simulink model "Grua"  (R2024b)
settings: Solver=VariableStepAuto  StartTime=0.0  StopTime=50.0  RelTol=1e-3
values from neighbouring files (symbols this model uses):
  A1 = [0 0 1 0; 0 0 0 1; 0 0 carrito_ss.A(2,2) 0; 0 pendulo_ss.A(2,1) 0 pendulo_ss.A(2,2)]    [Grua_Pendulo_Control.m]    (also in grua.mat = [0 0 0 0 0 0 0 -35.3130710133 1 0 -9.69067245938 0 ... (16 e)
  B1 = [0; pendulo_ss.B(1); carrito_ss.B(2); pendulo_ss.B(2)]    [Grua_Pendulo_Control.m]    (also in grua.mat = [0 -0.296894785399 0.236071876692 -1.46592019656])
  C = [1 0 0 0]    [Grua_Pendulo_Control.m]    (also in grua.mat)
  K = Ks(1:4)    [Grua_Pendulo_Control.m]    (also in grua.mat = [11.2779924086 -1.98610202692 -5.28014178733 -2.15028681626])
  K_q = Kq(1:4)    [Grua_Pendulo_Control.m]    (also in grua.mat = [50.0170795212 -5.53286476625 6.72231103684 -0.384358946683])
  Ki = -Ks(5)    [Grua_Pendulo_Control.m]    (also in grua.mat = 4.13832170273)
  Ki_q = -Kq(5)    [Grua_Pendulo_Control.m]    (also in grua.mat = 20)
libraries: simulink x5, slpidlib x3
settings Model: Creator=nagel  LastModifiedBy=nagel

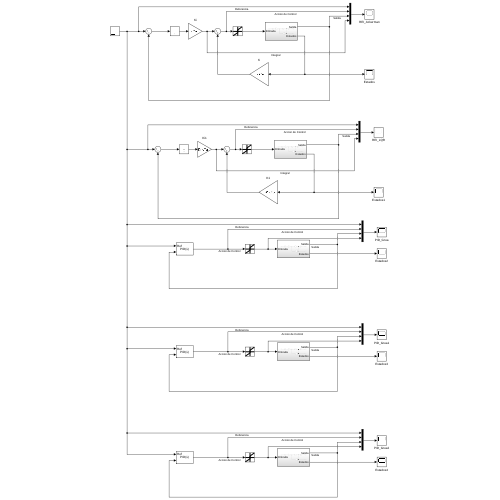
[thumbnail: Simulink's stored preview of the top-level diagram]
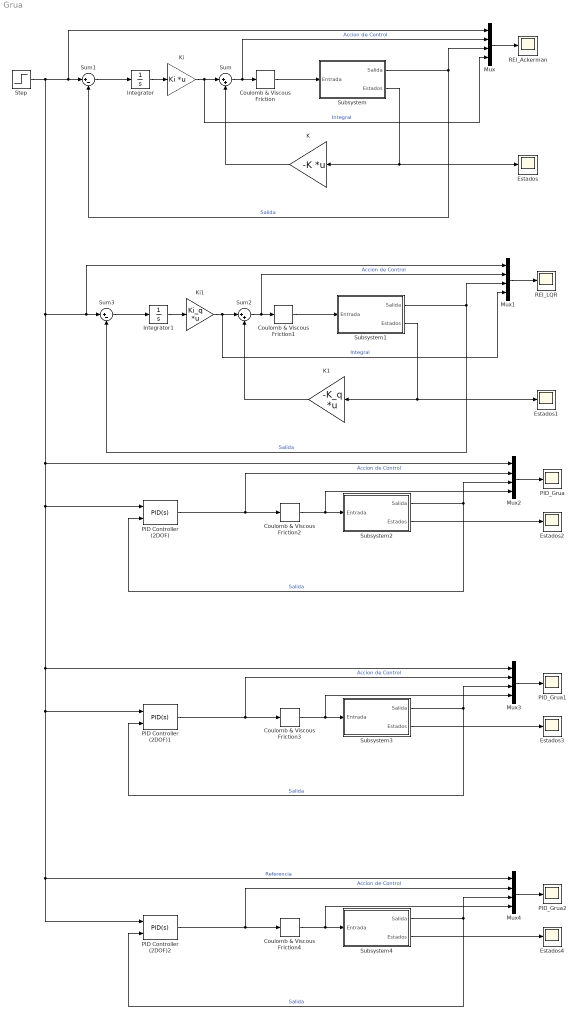
== system Grua ==
  Coulomb & Viscous Friction{,1..4} (5 alike) : simulink/Discontinuities/Coulomb & Viscous Friction  offset=[0.4]  gain=1
  Estados{,1..4} (5 alike) : Scope
  Integrator : Integrator
  Integrator1 : Integrator
  K : Gain  Gain=-K  Multiplication=Matrix(K*u)
  K1 : Gain  Gain=-K_q  Multiplication=Matrix(K*u)
  Ki : Gain  Gain=Ki  Multiplication=Matrix(K*u)
  Ki1 : Gain  Gain=Ki_q  Multiplication=Matrix(K*u)
  Mux{,1..4} (5 alike) : Mux
  PID Controller (2DOF) : slpidlib/PID Controller (2DOF)  Controller=PID  Form=Parallel  TimeDomain=Continuous-time  UseExternalTs=off  SampleTime=-1  IntegratorMethod=Forward Euler  FilterMethod=Forward Euler  ControllerParametersSource=internal  P=30.1626  I=0.3867  UseKiTs=off  D=0  UseExternalDerivativeSource=off  N=0  UseFilter=on  b=1  c=1  TunerSelectOption=Transfer Function Based (PID Tuner App)  InitialConditionSource=internal  InitialConditionForIntegrator=0  InitialConditionForFilter=0  DifferentiatorICPrevScaledInput=0  ExternalReset=none  TrackingMode=off  Kt=1  LimitOutput=off  SatLimitsSource=internal  UpperSaturationLimit=inf  LowerSaturationLimit=-inf  LinearizeAsGain=on  AntiWindupMode=none  Kb=1  LimitIntegrator=off  UpperIntegratorSaturationLimit=inf  LowerIntegratorSaturationLimit=-inf  POutMin=[]  POutMax=[]  IOutMin=[]  IOutMax=[]  DOutMin=[]  DOutMax=[]  NOutMin=[]  NOutMax=[]  bOutMin=[]  bOutMax=[]  cOutMin=[]  cOutMax=[]  SumOutMin=[]  SumOutMax=[]  SaturationOutMin=[]  SaturationOutMax=[]  PParamMin=[]  PParamMax=[]  IParamMin=[]  IParamMax=[]  DParamMin=[]  DParamMax=[]  NParamMin=[]  NParamMax=[]  bParamMin=[]  bParamMax=[]  cParamMin=[]  cParamMax=[]  KbParamMin=[]  KbParamMax=[]  KtParamMin=[]  KtParamMax=[]  KbOutMin=[]  KbOutMax=[]  KtOutMin=[]  KtOutMax=[]  IntegratorOutMin=[]  IntegratorOutMax=[]  FilterOutMin=[]  FilterOutMax=[]  SumI1OutMin=[]  SumI1OutMax=[]  SumI2OutMin=[]  SumI2OutMax=[]  SumI3OutMin=[]  SumI3OutMax=[]  SumI4OutMin=[]  SumI4OutMax=[]  SumDOutMin=[]  SumDOutMax=[]  Sum1OutMin=[]  Sum1OutMax=[]  Sum2OutMin=[]  Sum2OutMax=[]  Sum3OutMin=[]  Sum3OutMax=[]  DifferentiatorOutMin=[]  DifferentiatorOutMax=[]  FilterDiffOutCoefMin=[]  FilterDiffOutCoefMax=[]  ReciprocalOutMin=[]  ReciprocalOutMax=[]  SumDenOutMin=[]  SumDenOutMax=[]  SumNumOutMin=[]  SumNumOutMax=[]  DivideOutMin=[]  DivideOutMax=[]  UdiffTsProdOutMin=[]  UdiffTsProdOutMax=[]  NTsProdOutMin=[]  NTsProdOutMax=[]  UintegralTsProdOutMin=[]  UintegralTsProdOutMax=[]  UngainTsProdOutMin=[]  UngainTsProdOutMax=[]  ClampingZeroOutDataTypeStr=Inherit: Inherit via back propagation  ClampingZeroOutMin=[]  ClampingZeroOutMax=[]  FilterDenConstantOutDataTypeStr=Inherit: Inherit via back propagation  FilterDenConstantOutMin=[]  FilterDenConstantOutMax=[]  PCopyOutDataTypeStr=Inherit: Inherit via back propagation  PCopyOutMin=[]  PCopyOutMax=[]  NCopyOutDataTypeStr=Inherit: Inherit via back propagation  NCopyOutMin=[]  NCopyOutMax=[]  IntegratorContinuousStateAttributes=''  IntegratorStateMustResolveToSignalObject=off  IntegratorRTWStateStorageClass=Auto  FilterContinuousStateAttributes=''  FilterStateMustResolveToSignalObject=off  FilterRTWStateStorageClass=Auto  ParallelPVariant=InternalParameters  IdealPVariant=Disabled  IVariant=InternalParameters  DVariant=InternalParameters  bVariant=InternalParameters  cVariant=InternalParameters  IntegratorVariant=Continuous  SatVariant=Disabled  AWVariant=Passthrough  PCopyVariant=Disabled  TRVariant=Disabled  FdbkBlocksVariant=Forward  IdealPFdbkVariant=Disabled  SatFdbkVariant=Disabled  DerivativeFilterVariant=ContFilter  NVariant=InternalParameters  NCopyVariant=Disabled  FilterICVariant=InternalICsFilter  IntegratorICVariant=InternalICs  ExternalResetVariant=Disabled  TRSumVariant=Passthrough  SumFdbkVariant=Disabled  SumVariant=Sum_PID  TsampFilterVariant=InternalTs  TsampNgainVariant=Passthrough  TsampIntegralVariant=Disabled_SignalSpec  ExternalSaturationOutDataTypeStr=Inherit: Same as second input  DerivativeSourceVariant=ErrorSignal  PreIntVariant=InternalPreInt
  PID Controller (2DOF)1 : slpidlib/PID Controller (2DOF)  Controller=PID  Form=Parallel  TimeDomain=Continuous-time  UseExternalTs=off  SampleTime=-1  IntegratorMethod=Forward Euler  FilterMethod=Forward Euler  ControllerParametersSource=internal  P=16.75  I=95.23  UseKiTs=off  D=38.239  UseExternalDerivativeSource=off  N=270.27  UseFilter=on  b=1  c=1  TunerSelectOption=Transfer Function Based (PID Tuner App)  InitialConditionSource=internal  InitialConditionForIntegrator=0  InitialConditionForFilter=0  DifferentiatorICPrevScaledInput=0  ExternalReset=none  TrackingMode=off  Kt=1  LimitOutput=off  SatLimitsSource=internal  UpperSaturationLimit=inf  LowerSaturationLimit=-inf  LinearizeAsGain=on  AntiWindupMode=none  Kb=1  LimitIntegrator=off  UpperIntegratorSaturationLimit=inf  LowerIntegratorSaturationLimit=-inf  POutMin=[]  POutMax=[]  IOutMin=[]  IOutMax=[]  DOutMin=[]  DOutMax=[]  NOutMin=[]  NOutMax=[]  bOutMin=[]  bOutMax=[]  cOutMin=[]  cOutMax=[]  SumOutMin=[]  SumOutMax=[]  SaturationOutMin=[]  SaturationOutMax=[]  PParamMin=[]  PParamMax=[]  IParamMin=[]  IParamMax=[]  DParamMin=[]  DParamMax=[]  NParamMin=[]  NParamMax=[]  bParamMin=[]  bParamMax=[]  cParamMin=[]  cParamMax=[]  KbParamMin=[]  KbParamMax=[]  KtParamMin=[]  KtParamMax=[]  KbOutMin=[]  KbOutMax=[]  KtOutMin=[]  KtOutMax=[]  IntegratorOutMin=[]  IntegratorOutMax=[]  FilterOutMin=[]  FilterOutMax=[]  SumI1OutMin=[]  SumI1OutMax=[]  SumI2OutMin=[]  SumI2OutMax=[]  SumI3OutMin=[]  SumI3OutMax=[]  SumI4OutMin=[]  SumI4OutMax=[]  SumDOutMin=[]  SumDOutMax=[]  Sum1OutMin=[]  Sum1OutMax=[]  Sum2OutMin=[]  Sum2OutMax=[]  Sum3OutMin=[]  Sum3OutMax=[]  DifferentiatorOutMin=[]  DifferentiatorOutMax=[]  FilterDiffOutCoefMin=[]  FilterDiffOutCoefMax=[]  ReciprocalOutMin=[]  ReciprocalOutMax=[]  SumDenOutMin=[]  SumDenOutMax=[]  SumNumOutMin=[]  SumNumOutMax=[]  DivideOutMin=[]  DivideOutMax=[]  UdiffTsProdOutMin=[]  UdiffTsProdOutMax=[]  NTsProdOutMin=[]  NTsProdOutMax=[]  UintegralTsProdOutMin=[]  UintegralTsProdOutMax=[]  UngainTsProdOutMin=[]  UngainTsProdOutMax=[]  ClampingZeroOutDataTypeStr=Inherit: Inherit via back propagation  ClampingZeroOutMin=[]  ClampingZeroOutMax=[]  FilterDenConstantOutDataTypeStr=Inherit: Inherit via back propagation  FilterDenConstantOutMin=[]  FilterDenConstantOutMax=[]  PCopyOutDataTypeStr=Inherit: Inherit via back propagation  PCopyOutMin=[]  PCopyOutMax=[]  NCopyOutDataTypeStr=Inherit: Inherit via back propagation  NCopyOutMin=[]  NCopyOutMax=[]  IntegratorContinuousStateAttributes=''  IntegratorStateMustResolveToSignalObject=off  IntegratorRTWStateStorageClass=Auto  FilterContinuousStateAttributes=''  FilterStateMustResolveToSignalObject=off  FilterRTWStateStorageClass=Auto  ParallelPVariant=InternalParameters  IdealPVariant=Disabled  IVariant=InternalParameters  DVariant=InternalParameters  bVariant=InternalParameters  cVariant=InternalParameters  IntegratorVariant=Continuous  SatVariant=Disabled  AWVariant=Passthrough  PCopyVariant=Disabled  TRVariant=Disabled  FdbkBlocksVariant=Forward  IdealPFdbkVariant=Disabled  SatFdbkVariant=Disabled  DerivativeFilterVariant=ContFilter  NVariant=InternalParameters  NCopyVariant=Disabled  FilterICVariant=InternalICsFilter  IntegratorICVariant=InternalICs  ExternalResetVariant=Disabled  TRSumVariant=Passthrough  SumFdbkVariant=Disabled  SumVariant=Sum_PID  TsampFilterVariant=InternalTs  TsampNgainVariant=Passthrough  TsampIntegralVariant=Disabled_SignalSpec  ExternalSaturationOutDataTypeStr=Inherit: Same as second input  DerivativeSourceVariant=ErrorSignal  PreIntVariant=InternalPreInt
  PID Controller (2DOF)2 : slpidlib/PID Controller (2DOF)  Controller=PID  Form=Parallel  TimeDomain=Continuous-time  UseExternalTs=off  SampleTime=-1  IntegratorMethod=Forward Euler  FilterMethod=Forward Euler  ControllerParametersSource=internal  P=28  I=0  UseKiTs=off  D=0  UseExternalDerivativeSource=off  N=0  UseFilter=on  b=1  c=1  TunerSelectOption=Transfer Function Based (PID Tuner App)  InitialConditionSource=internal  InitialConditionForIntegrator=0  InitialConditionForFilter=0  DifferentiatorICPrevScaledInput=0  ExternalReset=none  TrackingMode=off  Kt=1  LimitOutput=off  SatLimitsSource=internal  UpperSaturationLimit=inf  LowerSaturationLimit=-inf  LinearizeAsGain=on  AntiWindupMode=none  Kb=1  LimitIntegrator=off  UpperIntegratorSaturationLimit=inf  LowerIntegratorSaturationLimit=-inf  POutMin=[]  POutMax=[]  IOutMin=[]  IOutMax=[]  DOutMin=[]  DOutMax=[]  NOutMin=[]  NOutMax=[]  bOutMin=[]  bOutMax=[]  cOutMin=[]  cOutMax=[]  SumOutMin=[]  SumOutMax=[]  SaturationOutMin=[]  SaturationOutMax=[]  PParamMin=[]  PParamMax=[]  IParamMin=[]  IParamMax=[]  DParamMin=[]  DParamMax=[]  NParamMin=[]  NParamMax=[]  bParamMin=[]  bParamMax=[]  cParamMin=[]  cParamMax=[]  KbParamMin=[]  KbParamMax=[]  KtParamMin=[]  KtParamMax=[]  KbOutMin=[]  KbOutMax=[]  KtOutMin=[]  KtOutMax=[]  IntegratorOutMin=[]  IntegratorOutMax=[]  FilterOutMin=[]  FilterOutMax=[]  SumI1OutMin=[]  SumI1OutMax=[]  SumI2OutMin=[]  SumI2OutMax=[]  SumI3OutMin=[]  SumI3OutMax=[]  SumI4OutMin=[]  SumI4OutMax=[]  SumDOutMin=[]  SumDOutMax=[]  Sum1OutMin=[]  Sum1OutMax=[]  Sum2OutMin=[]  Sum2OutMax=[]  Sum3OutMin=[]  Sum3OutMax=[]  DifferentiatorOutMin=[]  DifferentiatorOutMax=[]  FilterDiffOutCoefMin=[]  FilterDiffOutCoefMax=[]  ReciprocalOutMin=[]  ReciprocalOutMax=[]  SumDenOutMin=[]  SumDenOutMax=[]  SumNumOutMin=[]  SumNumOutMax=[]  DivideOutMin=[]  DivideOutMax=[]  UdiffTsProdOutMin=[]  UdiffTsProdOutMax=[]  NTsProdOutMin=[]  NTsProdOutMax=[]  UintegralTsProdOutMin=[]  UintegralTsProdOutMax=[]  UngainTsProdOutMin=[]  UngainTsProdOutMax=[]  ClampingZeroOutDataTypeStr=Inherit: Inherit via back propagation  ClampingZeroOutMin=[]  ClampingZeroOutMax=[]  FilterDenConstantOutDataTypeStr=Inherit: Inherit via back propagation  FilterDenConstantOutMin=[]  FilterDenConstantOutMax=[]  PCopyOutDataTypeStr=Inherit: Inherit via back propagation  PCopyOutMin=[]  PCopyOutMax=[]  NCopyOutDataTypeStr=Inherit: Inherit via back propagation  NCopyOutMin=[]  NCopyOutMax=[]  IntegratorContinuousStateAttributes=''  IntegratorStateMustResolveToSignalObject=off  IntegratorRTWStateStorageClass=Auto  FilterContinuousStateAttributes=''  FilterStateMustResolveToSignalObject=off  FilterRTWStateStorageClass=Auto  ParallelPVariant=InternalParameters  IdealPVariant=Disabled  IVariant=InternalParameters  DVariant=InternalParameters  bVariant=InternalParameters  cVariant=InternalParameters  IntegratorVariant=Continuous  SatVariant=Disabled  AWVariant=Passthrough  PCopyVariant=Disabled  TRVariant=Disabled  FdbkBlocksVariant=Forward  IdealPFdbkVariant=Disabled  SatFdbkVariant=Disabled  DerivativeFilterVariant=ContFilter  NVariant=InternalParameters  NCopyVariant=Disabled  FilterICVariant=InternalICsFilter  IntegratorICVariant=InternalICs  ExternalResetVariant=Disabled  TRSumVariant=Passthrough  SumFdbkVariant=Disabled  SumVariant=Sum_PID  TsampFilterVariant=InternalTs  TsampNgainVariant=Passthrough  TsampIntegralVariant=Disabled_SignalSpec  ExternalSaturationOutDataTypeStr=Inherit: Same as second input  DerivativeSourceVariant=ErrorSignal  PreIntVariant=InternalPreInt
  PID_Grua : Scope
  PID_Grua1 : Scope
  PID_Grua2 : Scope
  REI_Ackerman : Scope
  REI_LQR : Scope
  Step : Step  After=0.5  SampleTime=0
  Subsystem : Subsystem
  Subsystem1 : Subsystem
  Subsystem2 : Subsystem
  Subsystem3 : Subsystem
  Subsystem4 : Subsystem
  Sum : Sum  Inputs=|++
  Sum1 : Sum  Inputs=|+-
  Sum2 : Sum  Inputs=|++
  Sum3 : Sum  Inputs=|+-
  wires:
  Subsystem/1(Salida) -> Sum1/2, Mux/3  "Salida"
  Coulomb & Viscous Friction/1 -> Subsystem/1(Entrada)
  Subsystem/2(Estados) -> K/1, Estados/1
  Sum/1 -> Mux/2, Coulomb & Viscous Friction/1  "Accion de Control"
  K/1 -> Sum/2
  Integrator/1 -> Ki/1
  Ki/1 -> Mux/4, Sum/1  "Integral"
  Sum1/1 -> Integrator/1
  Mux/1 -> REI_Ackerman/1
  Sum2/1 -> Mux1/2, Coulomb & Viscous Friction1/1  "Accion de Control"
  Integrator1/1 -> Ki1/1
  K1/1 -> Sum2/2
  Sum3/1 -> Integrator1/1
  Mux1/1 -> REI_LQR/1
  Ki1/1 -> Mux1/4, Sum2/1  "Integral"
  Subsystem1/2(Estados) -> K1/1, Estados1/1
  Coulomb & Viscous Friction1/1 -> Subsystem1/1(Entrada)
  Subsystem1/1(Salida) -> Sum3/2, Mux1/3  "Salida"
  Subsystem2/2(Estados) -> Estados2/1
  Coulomb & Viscous Friction2/1 -> Mux2/4, Subsystem2/1(Entrada)
  PID Controller (2DOF)/1 -> Coulomb & Viscous Friction2/1, Mux2/2  "Accion de Control"
  Mux2/1 -> PID_Grua/1
  Subsystem2/1(Salida) -> Mux2/3, PID Controller (2DOF)/2  "Salida"
  Mux3/1 -> PID_Grua1/1
  Subsystem3/2(Estados) -> Estados3/1
  PID Controller (2DOF)1/1 -> Coulomb & Viscous Friction3/1, Mux3/2  "Accion de Control"
  Coulomb & Viscous Friction3/1 -> Mux3/4, Subsystem3/1(Entrada)
  Subsystem3/1(Salida) -> Mux3/3, PID Controller (2DOF)1/2  "Salida"
  Subsystem4/1(Salida) -> Mux4/3, PID Controller (2DOF)2/2  "Salida"
  Coulomb & Viscous Friction4/1 -> Mux4/4, Subsystem4/1(Entrada)
  PID Controller (2DOF)2/1 -> Coulomb & Viscous Friction4/1, Mux4/2  "Accion de Control"
  Subsystem4/2(Estados) -> Estados4/1
  Step/1 -> PID Controller (2DOF)2/1, Mux4/1, PID Controller (2DOF)1/1, Mux3/1, PID Controller (2DOF)/1, Mux2/1, Mux1/1, Sum3/1, Mux/1, Sum1/1  "Referencia"
  Mux4/1 -> PID_Grua2/1

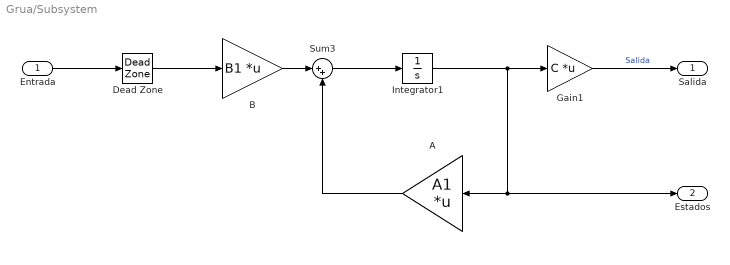
== system Grua/Subsystem ==
  Entrada : Inport
  A : Gain  Gain=A1  Multiplication=Matrix(K*u)
  B : Gain  Gain=B1  Multiplication=Matrix(K*u)
  Dead Zone : DeadZone  UpperValue=0.6
  Gain1 : Gain  Gain=C  Multiplication=Matrix(K*u)
  Integrator1 : Integrator
  Sum3 : Sum  Inputs=|++
  Salida : Outport
  Estados : Outport  Port=2
  wires:
  Sum3/1 -> Integrator1/1
  B/1 -> Sum3/1
  A/1 -> Sum3/2
  Gain1/1 -> Salida/1  "Salida"
  Integrator1/1 -> A/1, Estados/1, Gain1/1
  Entrada/1 -> Dead Zone/1
  Dead Zone/1 -> B/1

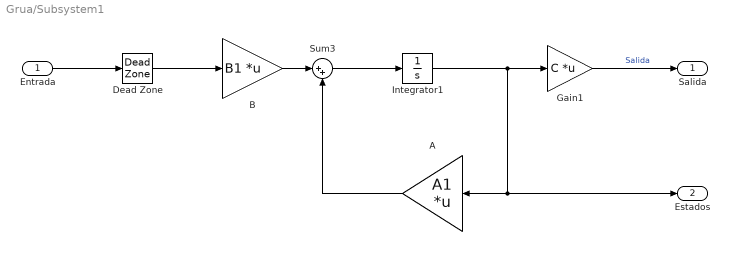
== system Grua/Subsystem1 ==
  Entrada : Inport
  A : Gain  Gain=A1  Multiplication=Matrix(K*u)
  B : Gain  Gain=B1  Multiplication=Matrix(K*u)
  Dead Zone : DeadZone  UpperValue=0.6
  Gain1 : Gain  Gain=C  Multiplication=Matrix(K*u)
  Integrator1 : Integrator
  Sum3 : Sum  Inputs=|++
  Salida : Outport
  Estados : Outport  Port=2
  wires:
  Sum3/1 -> Integrator1/1
  B/1 -> Sum3/1
  A/1 -> Sum3/2
  Gain1/1 -> Salida/1  "Salida"
  Integrator1/1 -> A/1, Estados/1, Gain1/1
  Entrada/1 -> Dead Zone/1
  Dead Zone/1 -> B/1

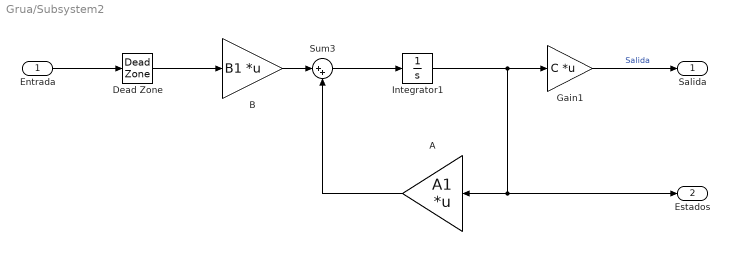
== system Grua/Subsystem2 ==
  Entrada : Inport
  A : Gain  Gain=A1  Multiplication=Matrix(K*u)
  B : Gain  Gain=B1  Multiplication=Matrix(K*u)
  Dead Zone : DeadZone  UpperValue=0.6
  Gain1 : Gain  Gain=C  Multiplication=Matrix(K*u)
  Integrator1 : Integrator
  Sum3 : Sum  Inputs=|++
  Salida : Outport
  Estados : Outport  Port=2
  wires:
  Sum3/1 -> Integrator1/1
  B/1 -> Sum3/1
  A/1 -> Sum3/2
  Gain1/1 -> Salida/1  "Salida"
  Integrator1/1 -> A/1, Estados/1, Gain1/1
  Entrada/1 -> Dead Zone/1
  Dead Zone/1 -> B/1

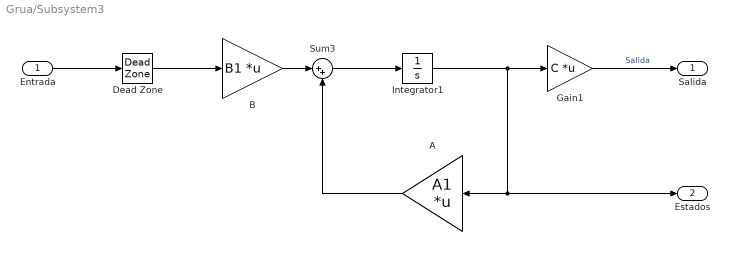
== system Grua/Subsystem3 ==
  Entrada : Inport
  A : Gain  Gain=A1  Multiplication=Matrix(K*u)
  B : Gain  Gain=B1  Multiplication=Matrix(K*u)
  Dead Zone : DeadZone  UpperValue=0.6
  Gain1 : Gain  Gain=C  Multiplication=Matrix(K*u)
  Integrator1 : Integrator
  Sum3 : Sum  Inputs=|++
  Salida : Outport
  Estados : Outport  Port=2
  wires:
  Sum3/1 -> Integrator1/1
  B/1 -> Sum3/1
  A/1 -> Sum3/2
  Gain1/1 -> Salida/1  "Salida"
  Integrator1/1 -> A/1, Estados/1, Gain1/1
  Entrada/1 -> Dead Zone/1
  Dead Zone/1 -> B/1

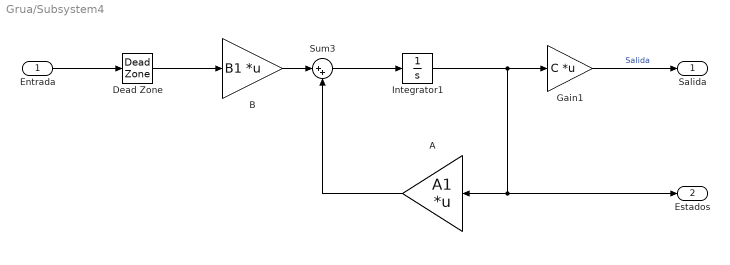
== system Grua/Subsystem4 ==
  Entrada : Inport
  A : Gain  Gain=A1  Multiplication=Matrix(K*u)
  B : Gain  Gain=B1  Multiplication=Matrix(K*u)
  Dead Zone : DeadZone  UpperValue=0.6
  Gain1 : Gain  Gain=C  Multiplication=Matrix(K*u)
  Integrator1 : Integrator
  Sum3 : Sum  Inputs=|++
  Salida : Outport
  Estados : Outport  Port=2
  wires:
  Sum3/1 -> Integrator1/1
  B/1 -> Sum3/1
  A/1 -> Sum3/2
  Gain1/1 -> Salida/1  "Salida"
  Integrator1/1 -> A/1, Estados/1, Gain1/1
  Entrada/1 -> Dead Zone/1
  Dead Zone/1 -> B/1
